simulink library "lib_Convection_SiederTate"  (R2015a)
settings: Solver=ode45  StartTime=0.0  StopTime=10.0  RelTol=1e-3
libraries: simulink x3
settings Model: Creator=jlkratz  LastModifiedBy=jlkratz

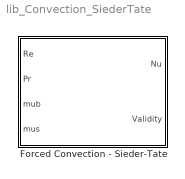
== system lib_Convection_SiederTate ==
  Forced Convection - Sieder-Tate : Subsystem
      mask help:
      | The block approximates the local Nusselt number for fully developed turbulent flow in a smooth circular tube using the Sieder-Tate correlation. For tubes with different shaped cross-sections this correlation can be used as a first approximation with the hydraulic diameter of the tube used in place of the tube diameter. The equation attempts to account for variations in thermal properties of the fluid which is mainly done through considering the viscosity of the fluid at the mean fluid temperature and at the tube surface temperature. This block is recommended more so than the Dittus-Boelter equation when the variation in temperature between the surface of the pipe and the bulk fluid is large. Restrictions to this correlation include:
      |
      | 0.7 <= Pr <= 16700
      | Re >= 10000
      | L/D >= 10 (L/D = entrance length / diameter) <-- fully developed
      |
      | This correlation is a good approxiamtion for uniform surface temperature and heat flux conditions.
      mask Help: web(which('Convection_TSAT_SiederTate.html'),'-helpbrowser')

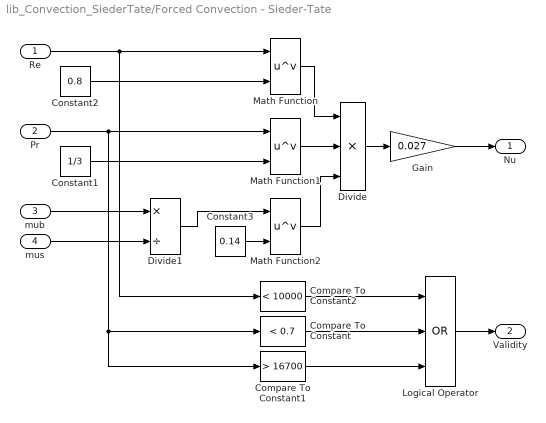
== system lib_Convection_SiederTate/Forced Convection - Sieder-Tate ==
  Re : Inport
  Pr : Inport  Port=2
  mub : Inport  Port=3
  mus : Inport  Port=4
  Compare To Constant : simulink/Logic and Bit Operations/Compare To Constant  relop=<  const=0.7  OutDataTypeStr=boolean
  Compare To Constant1 : simulink/Logic and Bit Operations/Compare To Constant  relop=>  const=16700  OutDataTypeStr=boolean
  Compare To Constant2 : simulink/Logic and Bit Operations/Compare To Constant  relop=<  const=10000  OutDataTypeStr=boolean
  Constant1 : Constant  Value=1/3
  Constant2 : Constant  Value=0.8
  Constant3 : Constant  Value=0.14
  Divide : Product  Inputs=***
  Divide1 : Product  Inputs=*/
  Gain : Gain  Gain=0.027
  Logical Operator : Logic  Operator=OR  Inputs=3  AllPortsSameDT=off  OutDataTypeStr=boolean
  Math Function : Math  Operator=pow  SaturateOnIntegerOverflow=on
  Math Function1 : Math  Operator=pow  SaturateOnIntegerOverflow=on
  Math Function2 : Math  Operator=pow  SaturateOnIntegerOverflow=on
  Nu : Outport
  Validity : Outport  Port=2
  wires:
  Math Function2/1 -> Divide/3
  Constant3/1 -> Math Function2/2
  Divide1/1 -> Math Function2/1
  mus/1 -> Divide1/2
  mub/1 -> Divide1/1
  Constant1/1 -> Math Function1/2
  Gain/1 -> Nu/1
  Pr/1 -> Math Function1/1, Compare To Constant1/1, Compare To Constant/1
  Math Function/1 -> Divide/1
  Divide/1 -> Gain/1
  Re/1 -> Compare To Constant2/1, Math Function/1
  Compare To Constant1/1 -> Logical Operator/3
  Logical Operator/1 -> Validity/1
  Compare To Constant/1 -> Logical Operator/2
  Compare To Constant2/1 -> Logical Operator/1
  Math Function1/1 -> Divide/2
  Constant2/1 -> Math Function/2
